simulink model "sampleModel225"  (R2021b)
settings: Solver=VariableStepAuto  StartTime=0.0  StopTime=10.0  RelTol=1e-3
undefined symbols (not defined in the file or in its folder): DiscIntNeverNeededParam, Newton, Raphson
libraries: simulink x4, slpidlib x1
settings Model: Creator=user  LastModifiedBy=user

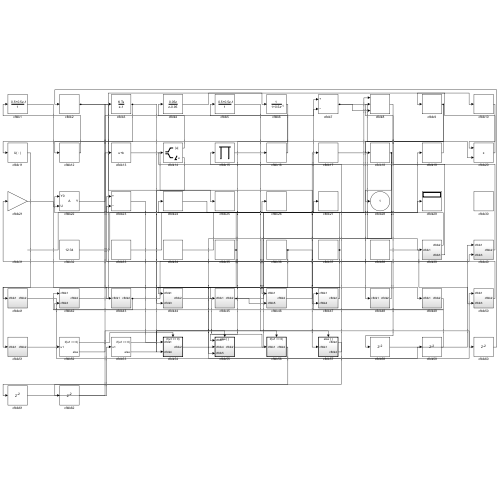
[thumbnail: Simulink's stored preview of the top-level diagram]
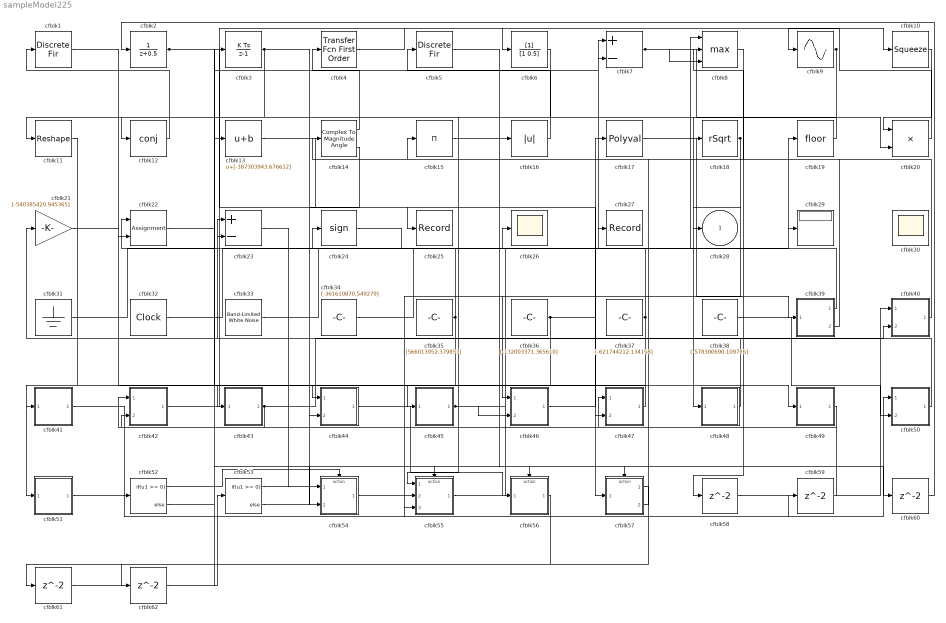
== system sampleModel225 ==
  cfblk1 : DiscreteFir  SampleTime=1
  cfblk10 : Squeeze
  cfblk11 : Reshape
  cfblk12 : Math  Operator=conj  SaturateOnIntegerOverflow=on
  cfblk13 : Bias  Bias=[-387303943.676612]
  cfblk14 : ComplexToMagnitudeAngle
  cfblk15 : Product  Inputs=*
  cfblk16 : Abs
  cfblk17 : Polyval  Coefs=[ +2.081618890e-019, -1.441693666e-014, +4.719686976e-010, -8.536869453e-006, +1.621573104e-001, -8.087801117e+001 ]
  cfblk18 : Sqrt  Operator=rSqrt  AlgorithmType=Newton-Raphson  SaturateOnIntegerOverflow=on
  cfblk19 : Rounding
  cfblk2 : DiscreteTransferFcn  SampleTime=1
  cfblk20 : Product
  cfblk21 : Gain  Gain=[-540385420.945365]
  cfblk22 : Assignment  DiagnosticForDimensions=Warning  IndexOptions=Index vector (dialog)  Indices=1  OutputSizes=1
  cfblk23 : Sum  Inputs=+-
  cfblk24 : Signum
  cfblk25 : Record  FileSettingsInternal="{\"entries\":[{\"content\":{\"excelSettings\":{\"content\":{},\"type\":\"Streamout.ExcelSettings\"}},\"type\":\"Streamout.FileSettingStorage\",\"uuid\":\"4e7e3b95-72b2-4485-886b-8d009dfdaece\"}],\"packageUris\":[\"http://schema.mathworks.com/mf0/streamout_blocks/R2020a\"],\"version\":\"1.0\"}"  SignalsInternal="{\"entries\":[{\"content\":{\"signals\":[{\"content\":{\"blockPath\":[\"sampleModel225/cfblk25\"],\"channel\":[],\"dimensions\":[1],\"domain\":\"sampleModel225/cfblk25\",\"lineColor\":\"#edb120\",\"plots\":[1],\"port\":1,\"sid\":[\"\"],\"signalID\":8807,\"signalName\":\"cfblk2\"},\"type\":\"RecordBlkView.Signal\",\"uuid\":\"caa7a7fe-cf03-4d92-84b3-6ee960b38914\"}]},\"type\":\"RecordBlkView.InputSignals\",\"uuid\":\"f0579e01-41f7-419e-960d-229318a79fff\"}],\"packageUris\":[\"http://schema.mathworks.com/mf0/streamout_blocks/R2020a\"],\"version\":\"1.0\"}"  VisualizationBindings="{\"sparklinesplugin\":{\"info\":[{\"bindingParametersList\":[],\"subplotID\":1}]}}"
  cfblk26 : Scope
  cfblk27 : Record  FileSettingsInternal="{\"entries\":[{\"content\":{\"excelSettings\":{\"content\":{},\"type\":\"Streamout.ExcelSettings\"}},\"type\":\"Streamout.FileSettingStorage\",\"uuid\":\"49384f4d-e1c6-4fc9-897d-458b70a04d99\"}],\"packageUris\":[\"http://schema.mathworks.com/mf0/streamout_blocks/R2020a\"],\"version\":\"1.0\"}"  SignalsInternal="{\"entries\":[{\"content\":{\"signals\":[{\"content\":{\"blockPath\":[\"sampleModel225/cfblk27\"],\"channel\":[],\"dimensions\":[1],\"domain\":\"sampleModel225/cfblk27\",\"lineColor\":\"#7e2f8e\",\"plots\":[1],\"port\":1,\"sid\":[\"\"],\"signalID\":8811,\"signalName\":\"cfblk34\"},\"type\":\"RecordBlkView.Signal\",\"uuid\":\"c564fc10-3473-46ad-84b2-5b0f433de686\"}]},\"type\":\"RecordBlkView.InputSignals\",\"uuid\":\"7b61474a-02df-4bbb-8ab8-049155fb11e6\"}],\"packageUris\":[\"http://schema.mathworks.com/mf0/streamout_blocks/R2020a\"],\"version\":\"1.0\"}"  VisualizationBindings="{\"sparklinesplugin\":{\"info\":[{\"bindingParametersList\":[],\"subplotID\":1}]}}"
  cfblk29 : Display
  cfblk3 : DiscreteIntegrator  ICPrevOutput=DiscIntNeverNeededParam  ICPrevScaledInput=DiscIntNeverNeededParam
  cfblk30 : Scope
      settings: Floating=on
  cfblk31 : Ground
  cfblk32 : DigitalClock
  cfblk33 : simulink/Sources/Band-Limited White Noise  Cov=[6115807268.208452]  Ts=0.1  seed=[1507907618.000000]
  cfblk34 : Constant  Value=[-361610870.549279]  SampleTime=1
  cfblk35 : Constant  Value=[566013952.379853]  SampleTime=1
  cfblk36 : Constant  Value=[-132003371.365610]  SampleTime=1
  cfblk37 : Constant  Value=[-621744212.134158]  SampleTime=1
  cfblk38 : Constant  Value=[-578300690.109726]  SampleTime=1
  cfblk39 : Subsystem
  cfblk4 : simulink/Discrete/Transfer Fcn First Order  PoleZ=0.95  ICPrevOutput=0.0  DoSatur=off
  cfblk40 : Subsystem
  cfblk41 : Subsystem
  cfblk42 : Subsystem
  cfblk43 : Subsystem
  cfblk44 : Subsystem
  cfblk45 : Subsystem
  cfblk46 : Subsystem
  cfblk47 : Subsystem
  cfblk48 : Subsystem
  cfblk49 : Subsystem
  cfblk5 : DiscreteFir  SampleTime=1
  cfblk50 : Subsystem
  cfblk51 : Subsystem
  cfblk52 : If  IfExpression=u1 >= 0  SampleTime=1
  cfblk53 : If  IfExpression=u1 >= 0  SampleTime=1
  cfblk54 : Subsystem  TreatAsAtomicUnit=on
  cfblk55 : Subsystem  TreatAsAtomicUnit=on
  cfblk56 : Subsystem  TreatAsAtomicUnit=on
  cfblk57 : Subsystem  TreatAsAtomicUnit=on
  cfblk{58..62} (5 alike) : Delay  SampleTime=1
  cfblk6 : DiscreteFilter  SampleTime=1
  cfblk7 : Sum  Inputs=+-
  cfblk8 : MinMax  Function=max  Inputs=3
  cfblk9 : Sin  TimeSource=Use external signal  SampleTime=0
  cfblk28 : Outport
  wires:
  cfblk23/1 -> cfblk54/1(cfblk1)
  cfblk9/1 -> cfblk48/1(cfblk1), cfblk55/1(cfblk1)
  cfblk16/1 -> cfblk5/1
  cfblk42/1(cfblk2) -> cfblk6/1
  cfblk41/1(cfblk2) -> cfblk50/1(cfblk1)
  cfblk35/1 -> cfblk51/1(cfblk1), cfblk23/2
  cfblk38/1 -> cfblk50/2(cfblk3)
  cfblk2/1 -> cfblk25/1, cfblk45/1(cfblk1)
  cfblk48/1(cfblk2) -> cfblk21/1
  cfblk17/1 -> cfblk39/1(cfblk1)
  cfblk19/1 -> cfblk18/1
  cfblk20/1 -> cfblk9/1
  cfblk18/1 -> cfblk28/1, cfblk46/1(cfblk1), cfblk55/2(cfblk4)
  cfblk24/1 -> cfblk26/1
  cfblk15/1 -> cfblk16/1
  cfblk4/1 -> cfblk10/1
  cfblk50/1(cfblk2) -> cfblk23/1
  cfblk33/1 -> cfblk19/1
  cfblk37/1 -> cfblk22/1, cfblk55/3(cfblk5)
  cfblk32/1 -> cfblk8/1
  cfblk39/1(cfblk2) -> cfblk24/1
  cfblk1/1 -> cfblk22/2
  cfblk6/1 -> cfblk11/1
  cfblk10/1 -> cfblk20/1
  cfblk55/1(cfblk2) -> cfblk29/1
  cfblk7/1 -> cfblk20/2, cfblk8/3
  cfblk49/1(cfblk2) -> cfblk47/1(cfblk1)
  cfblk14/1 -> cfblk4/1
  cfblk21/1 -> cfblk43/1(cfblk1)
  cfblk44/1(cfblk2) -> cfblk56/1(cfblk1)
  cfblk22/1 -> cfblk7/1
  cfblk31/1 -> cfblk13/1
  cfblk43/1(cfblk2) -> cfblk40/2(cfblk3), cfblk42/2(cfblk3)
  cfblk47/1(cfblk2) -> cfblk44/1(cfblk1)
  cfblk14/2 -> cfblk54/2(cfblk4)
  cfblk13/1 -> cfblk57/1(cfblk1)
  cfblk12/1 -> cfblk1/1
  cfblk36/1 -> cfblk47/2(cfblk4), cfblk44/2(cfblk3)
  cfblk45/1(cfblk2) -> cfblk7/2, cfblk46/2(cfblk5)
  cfblk46/1(cfblk2) -> cfblk17/1
  cfblk39/2(cfblk3) -> cfblk15/1
  cfblk34/1 -> cfblk27/1
  cfblk3/1 -> cfblk49/1(cfblk1), cfblk12/1
  cfblk40/1(cfblk2) -> cfblk8/2
  cfblk51/1(cfblk2) -> cfblk52/1
  cfblk57/2(cfblk4) -> cfblk14/1
  cfblk11/1 -> cfblk41/1(cfblk1)
  cfblk52/1 -> cfblk54/Action
  cfblk52/2 -> cfblk55/Action
  cfblk53/1 -> cfblk56/Action
  cfblk53/2 -> cfblk57/Action
  cfblk8/1 -> cfblk58/1
  cfblk58/1 -> cfblk40/1(cfblk1)
  cfblk54/1(cfblk2) -> cfblk59/1
  cfblk59/1 -> cfblk42/1(cfblk1)
  cfblk5/1 -> cfblk60/1
  cfblk60/1 -> cfblk2/1
  cfblk56/1(cfblk2) -> cfblk61/1
  cfblk61/1 -> cfblk3/1
  cfblk57/1(cfblk2) -> cfblk62/1
  cfblk62/1 -> cfblk53/1

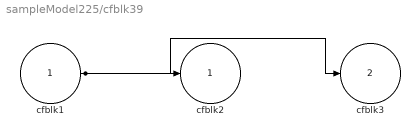
== system sampleModel225/cfblk39 ==
  cfblk1 : Inport
  cfblk2 : Outport
  cfblk3 : Outport  Port=2
  wires:
  cfblk1/1 -> cfblk3/1, cfblk2/1

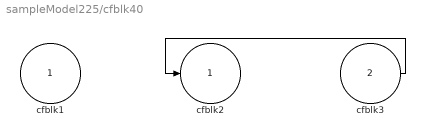
== system sampleModel225/cfblk40 ==
  cfblk1 : Inport
  cfblk3 : Inport  Port=2
  cfblk2 : Outport
  wires:
  cfblk3/1 -> cfblk2/1

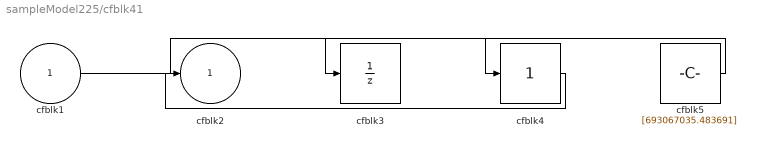
== system sampleModel225/cfblk41 ==
  cfblk1 : Inport
  cfblk3 : UnitDelay  HasFrameUpgradeWarning=on
  cfblk4 : simulink/Math Operations/Slider Gain  gain=1  low=0  high=2
  cfblk5 : Constant  Value=[693067035.483691]  SampleTime=1
  cfblk2 : Outport
  wires:
  cfblk1/1 -> cfblk4/1
  cfblk4/1 -> cfblk2/1
  cfblk5/1 -> cfblk3/1

== system sampleModel225/cfblk42 ==
  cfblk1 : Inport
  cfblk3 : Inport  Port=2
  cfblk2 : Outport
  wires:
  cfblk1/1 -> cfblk2/1

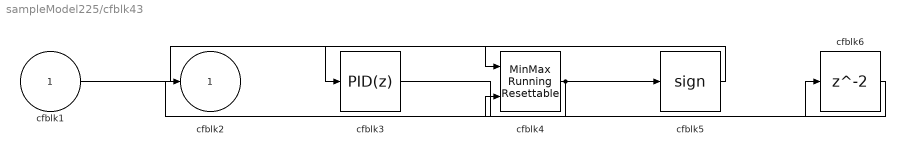
== system sampleModel225/cfblk43 ==
  cfblk1 : Inport
  cfblk3 : slpidlib/PID Controller  Controller=PID  Form=Parallel  TimeDomain=Discrete-time  UseExternalTs=off  SampleTime=1  IntegratorMethod=Forward Euler  FilterMethod=Forward Euler  ControllerParametersSource=internal  P=1  I=1  D=0  UseFilter=on  N=100  TunerSelectOption=Transfer Function Based (PID Tuner App)  InitialConditionSource=internal  InitialConditionForIntegrator=0  InitialConditionForFilter=0  DifferentiatorICPrevScaledInput=0  ExternalReset=none  TrackingMode=off  Kt=1  LimitOutput=off  SatLimitsSource=internal  UpperSaturationLimit=inf  LowerSaturationLimit=-inf  LinearizeAsGain=off  AntiWindupMode=none  Kb=1  POutMin=[]  POutMax=[]  IOutMin=[]  IOutMax=[]  DOutMin=[]  DOutMax=[]  NOutMin=[]  NOutMax=[]  SumOutMin=[]  SumOutMax=[]  SaturationOutMin=[]  SaturationOutMax=[]  PParamMin=[]  PParamMax=[]  IParamMin=[]  IParamMax=[]  DParamMin=[]  DParamMax=[]  NParamMin=[]  NParamMax=[]  KbParamMin=[]  KbParamMax=[]  KtParamMin=[]  KtParamMax=[]  KbOutMin=[]  KbOutMax=[]  KtOutMin=[]  KtOutMax=[]  IntegratorOutMin=[]  IntegratorOutMax=[]  FilterOutMin=[]  FilterOutMax=[]  SumI1OutMin=[]  SumI1OutMax=[]  SumI2OutMin=[]  SumI2OutMax=[]  SumI3OutMin=[]  SumI3OutMax=[]  SumI4OutMin=[]  SumI4OutMax=[]  SumDOutMin=[]  SumDOutMax=[]  DifferentiatorOutMin=[]  DifferentiatorOutMax=[]  FilterDiffOutCoefMin=[]  FilterDiffOutCoefMax=[]  ReciprocalOutMin=[]  ReciprocalOutMax=[]  SumDenOutMin=[]  SumDenOutMax=[]  SumNumOutMin=[]  SumNumOutMax=[]  DivideOutMin=[]  DivideOutMax=[]  UdiffTsProdOutMin=[]  UdiffTsProdOutMax=[]  NTsProdOutMin=[]  NTsProdOutMax=[]  UintegralTsProdOutMin=[]  UintegralTsProdOutMax=[]  UngainTsProdOutMin=[]  UngainTsProdOutMax=[]  IntegratorContinuousStateAttributes=''  IntegratorStateMustResolveToSignalObject=off  IntegratorRTWStateStorageClass=Auto  FilterContinuousStateAttributes=''  FilterStateMustResolveToSignalObject=off  FilterRTWStateStorageClass=Auto  ParallelPVariant=InternalParameters  IdealPVariant=Disabled  IVariant=InternalParameters  DVariant=InternalParameters  IntegratorVariant=Discrete  SatVariant=Disabled  AWVariant=Passthrough  PCopyVariant=Disabled  TRVariant=Disabled  FdbkBlocksVariant=Forward  IdealPFdbkVariant=Disabled  SatFdbkVariant=Disabled  DerivativeFilterVariant=ForwardEulerFilter  NVariant=InternalParameters  NCopyVariant=Disabled  FilterICVariant=InternalICsFilter  IntegratorICVariant=InternalICs  ExternalResetVariant=Disabled  TRSumVariant=Passthrough  SumFdbkVariant=Disabled  SumVariant=Sum_PID  TsampFilterVariant=InternalTs  TsampNgainVariant=Passthrough  TsampIntegralVariant=Passthrough  ExternalSaturationOutDataTypeStr=Inherit: Same as second input
  cfblk4 : simulink/Math Operations/MinMax Running Resettable  Function=min  vinit=0.0
  cfblk5 : Signum
  cfblk6 : Delay  SampleTime=1
  cfblk2 : Outport
  wires:
  cfblk1/1 -> cfblk4/1
  cfblk4/1 -> cfblk2/1, cfblk5/1
  cfblk5/1 -> cfblk3/1
  cfblk3/1 -> cfblk6/1
  cfblk6/1 -> cfblk4/2

== system sampleModel225/cfblk44 ==
  cfblk1 : Inport
  cfblk3 : Inport  Port=2
  cfblk2 : Outport
  wires:
  cfblk1/1 -> cfblk2/1

== system sampleModel225/cfblk45 ==
  cfblk1 : Inport
  cfblk3 : Constant  Value=[27250366.343216]  SampleTime=1
  cfblk2 : Outport
  wires:
  cfblk3/1 -> cfblk2/1

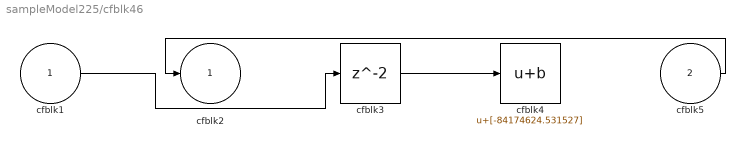
== system sampleModel225/cfblk46 ==
  cfblk1 : Inport
  cfblk5 : Inport  Port=2
  cfblk3 : Delay  SampleTime=1
  cfblk4 : Bias  Bias=[-84174624.531527]
  cfblk2 : Outport
  wires:
  cfblk3/1 -> cfblk4/1
  cfblk5/1 -> cfblk2/1
  cfblk1/1 -> cfblk3/1

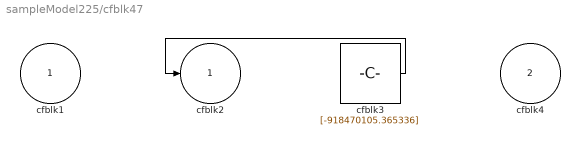
== system sampleModel225/cfblk47 ==
  cfblk1 : Inport
  cfblk4 : Inport  Port=2
  cfblk3 : Constant  Value=[-918470105.365336]  SampleTime=1
  cfblk2 : Outport
  wires:
  cfblk3/1 -> cfblk2/1

== system sampleModel225/cfblk48 ==
  cfblk1 : Inport
  cfblk3 : UnaryMinus
  cfblk2 : Outport
  wires:
  cfblk3/1 -> cfblk2/1
  cfblk1/1 -> cfblk3/1

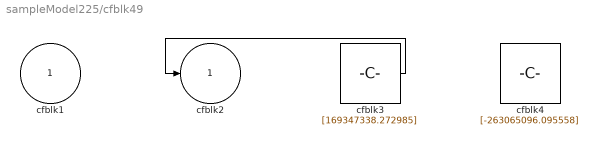
== system sampleModel225/cfblk49 ==
  cfblk1 : Inport
  cfblk3 : Constant  Value=[169347338.272985]  SampleTime=1
  cfblk4 : Constant  Value=[-263065096.095558]  SampleTime=1
  cfblk2 : Outport
  wires:
  cfblk3/1 -> cfblk2/1

== system sampleModel225/cfblk50 ==
  cfblk1 : Inport
  cfblk3 : Inport  Port=2
  cfblk2 : Outport
  wires:
  cfblk1/1 -> cfblk2/1

== system sampleModel225/cfblk51 ==
  cfblk1 : Inport
  cfblk3 : DiscreteIntegrator  ICPrevOutput=DiscIntNeverNeededParam  ICPrevScaledInput=DiscIntNeverNeededParam
  cfblk2 : Outport
  wires:
  cfblk1/1 -> cfblk3/1
  cfblk3/1 -> cfblk2/1

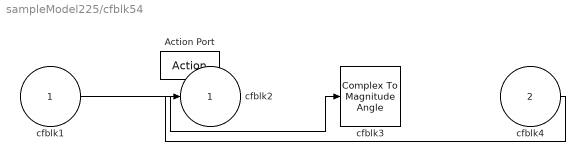
== system sampleModel225/cfblk54 ==
  cfblk1 : Inport
  cfblk4 : Inport  Port=2
  Action Port : ActionPort  ActionPortLabel=if(u1 >= 0)
  cfblk3 : ComplexToMagnitudeAngle
  cfblk2 : Outport
  wires:
  cfblk1/1 -> cfblk3/1
  cfblk4/1 -> cfblk2/1

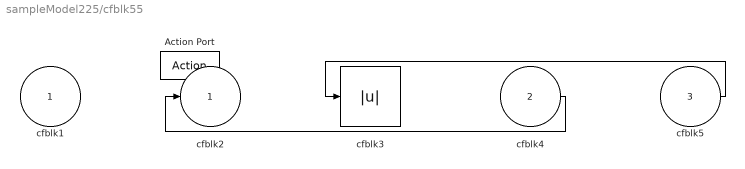
== system sampleModel225/cfblk55 ==
  cfblk1 : Inport
  cfblk4 : Inport  Port=2
  cfblk5 : Inport  Port=3
  Action Port : ActionPort  ActionPortLabel=else
  cfblk3 : Abs
  cfblk2 : Outport
  wires:
  cfblk5/1 -> cfblk3/1
  cfblk4/1 -> cfblk2/1

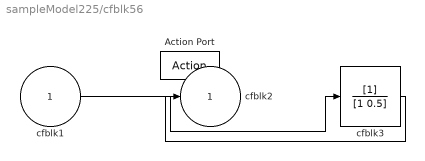
== system sampleModel225/cfblk56 ==
  cfblk1 : Inport
  Action Port : ActionPort  ActionPortLabel=if(u1 >= 0)
  cfblk3 : DiscreteFilter
  cfblk2 : Outport
  wires:
  cfblk1/1 -> cfblk3/1
  cfblk3/1 -> cfblk2/1

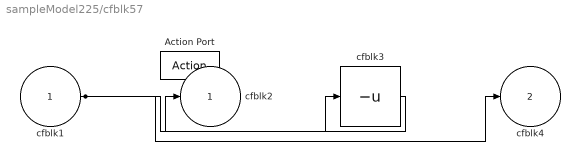
== system sampleModel225/cfblk57 ==
  cfblk1 : Inport
  Action Port : ActionPort  ActionPortLabel=else
  cfblk3 : UnaryMinus
  cfblk2 : Outport
  cfblk4 : Outport  Port=2
  wires:
  cfblk3/1 -> cfblk2/1
  cfblk1/1 -> cfblk4/1, cfblk3/1
